simulink model "bpsk_rx4"  (Simulink 8.5)
settings: Solver=FixedStepDiscrete  StartTime=0.0  StopTime=1000  RelTol=1e-3
libraries: dsp_blocks x8
settings Model: Creator=biruk  LastModifiedBy=biruk
settings DataIOCC: SignalLoggingSaveFormat=Dataset
settings OptimizationCC: ExpressionDepthLimit=128
settings DebuggingCC: UnderspecifiedInitializationDetection=Simplified  MergeDetectMultiDrivingBlocksExec=error  FcnCallInpInsideContextMsg=EnableAllAsError  StateNameClashWarn=none
settings GRTTargetCC: CombineOutputUpdateFcns=on  GRTInterface=off

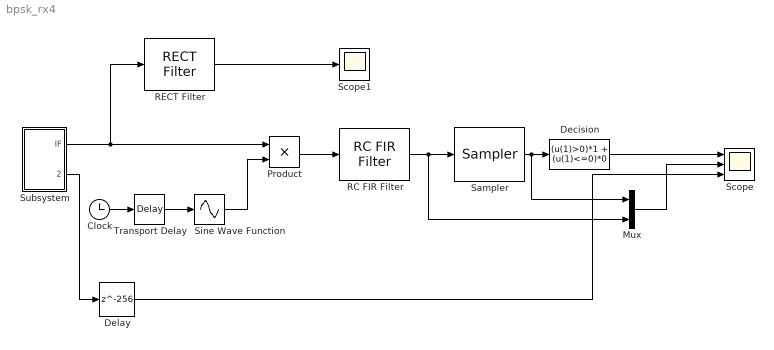
== system bpsk_rx4 ==
  Clock : Clock
  Decision : Fcn  Expr=(u(1)>0)*1 + (u(1)<=0)*0
  Delay : Delay  DelayLength=256
  Mux : Mux  Inputs=2
  Product : Product
  RC FIR Filter : dsp_blocks/Filters/RC FIR Filter  period=50  beta=0.5  root=on  filt_len=512  win_type=on
  RECT Filter : dsp_blocks/Filters/RECT Filter  f0=0.03  f1=0.07  filt_len=80
  Sampler : dsp_blocks/Conversions/Sampler  offset=512  samp_period=50
  Scope : Scope  NumInputPorts=3
      settings: TimeRange=2417.140996168582  YMin=-5~-0.9553072625698338~-5  YMax=5~0.8212290502793289~5
  Scope1 : Scope
  Sine Wave Function : Sin  TimeSource=Use external signal  Amplitude=2  Frequency=2*pi*0.1  SampleTime=0
  Subsystem : Subsystem
  Transport Delay : TransportDelay  DelayTime=4
  wires:
  Subsystem/1(IF) -> RECT Filter/1, Product/1
  Sine Wave Function/1 -> Product/2
  Product/1 -> RC FIR Filter/1
  RC FIR Filter/1 -> Mux/2, Sampler/1
  Sampler/1 -> Mux/1, Decision/1
  Subsystem/2("Debug ") -> Delay/1
  Decision/1 -> Scope/1
  Delay/1 -> Scope/3
  Mux/1 -> Scope/2
  Clock/1 -> Transport Delay/1
  Transport Delay/1 -> Sine Wave Function/1
  RECT Filter/1 -> Scope1/1

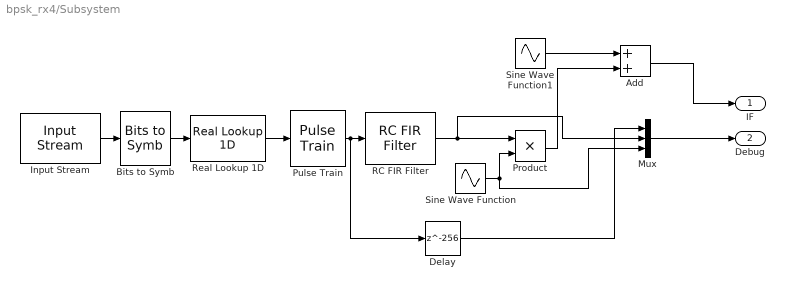
== system bpsk_rx4/Subsystem ==
  Add : Sum
  Bits to Symb : dsp_blocks/Conversions/Bits to Symb
  Delay : Delay  DelayLength=256
  Input Stream : dsp_blocks/Sources//Sinks/Input Stream  period=50  width=1  fname=rand.mat
  Mux : Mux  Inputs=3
  Product : Product
  Pulse Train : dsp_blocks/Conversions/Pulse Train  period=50
  RC FIR Filter : dsp_blocks/Filters/RC FIR Filter  period=50  beta=0.5  root=on  filt_len=512  win_type=on
  Real Lookup 1D : dsp_blocks/Conversions/Real Lookup 1D  table=[-1 1]
  Sine Wave Function : Sin  Frequency=2*pi*0.1  SampleTime=0
  Sine Wave Function1 : Sin  Amplitude=0.5  Frequency=2*pi*0.05  SampleTime=0
  IF : Outport
  "Debug " : Outport  Port=2
  wires:
  Sine Wave Function/1 -> Product/2, Mux/3
  Pulse Train/1 -> Delay/1, RC FIR Filter/1
  RC FIR Filter/1 -> Mux/2, Product/1
  Real Lookup 1D/1 -> Pulse Train/1
  Bits to Symb/1 -> Real Lookup 1D/1
  Input Stream/1 -> Bits to Symb/1
  Mux/1 -> "Debug "/1
  Delay/1 -> Mux/1
  Sine Wave Function1/1 -> Add/1
  Product/1 -> Add/2
  Add/1 -> IF/1
